simulink library "security_block"  (R2023b)
settings: Solver=VariableStepAuto  StartTime=0.0  StopTime=10.0  RelTol=1e-3
settings Model: Creator=mueller.chris-it22  LastModifiedBy=kilia

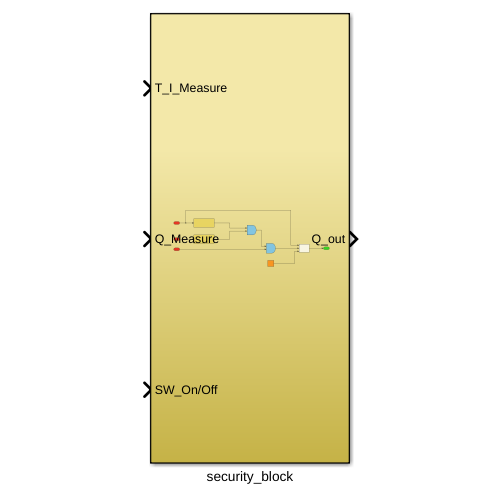
[thumbnail: Simulink's stored preview of the top-level diagram]
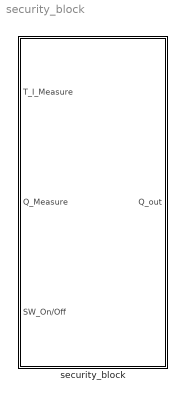
== system security_block ==
  security_block : Subsystem

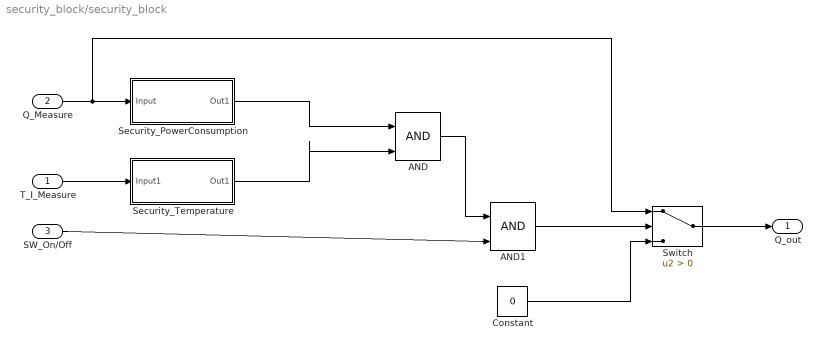
== system security_block/security_block ==
  T_I_Measure : Inport
  Q_Measure : Inport  Port=2
  SW_On/Off : Inport  Port=3
  AND : Logic  IconShape=distinctive  AllPortsSameDT=off  OutDataTypeStr=boolean
  AND1 : Logic  IconShape=distinctive  AllPortsSameDT=off  OutDataTypeStr=boolean
  Constant : Constant  Value=0
  Security_PowerConsumption : Subsystem
  Security_Temperature : Subsystem
  Switch : Switch  Criteria=u2 > Threshold  SaturateOnIntegerOverflow=off  InputSameDT=off
  Q_out : Outport
  wires:
  Q_Measure/1 -> Switch/1, Security_PowerConsumption/1(Input)
  T_I_Measure/1 -> Security_Temperature/1(Input1)
  Security_PowerConsumption/1(Out1) -> AND/1
  Security_Temperature/1(Out1) -> AND/2
  AND1/1 -> Switch/2
  SW_On/Off/1 -> AND1/2
  Switch/1 -> Q_out/1
  Constant/1 -> Switch/3
  AND/1 -> AND1/1

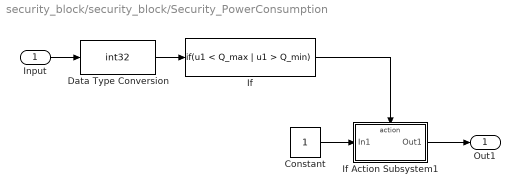
== system security_block/security_block/Security_PowerConsumption ==
  Input : Inport
  Constant : Constant
  Data Type Conversion : DataTypeConversion  OutDataTypeStr=int32  SaturateOnIntegerOverflow=off  RndMeth=Floor
  If : If  IfExpression=u1 < Q_max | u1 > Q_min  ShowElse=off
  If Action Subsystem1 : Subsystem  TreatAsAtomicUnit=on
  Out1 : Outport
  wires:
  Input/1 -> Data Type Conversion/1
  If/1 -> If Action Subsystem1/Action
  If Action Subsystem1/1(Out1) -> Out1/1
  Constant/1 -> If Action Subsystem1/1(In1)
  Data Type Conversion/1 -> If/1

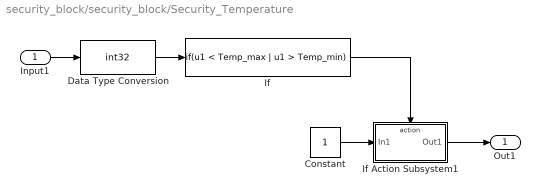
== system security_block/security_block/Security_Temperature ==
  Input1 : Inport
  Constant : Constant
  Data Type Conversion : DataTypeConversion  OutDataTypeStr=int32  SaturateOnIntegerOverflow=off  RndMeth=Floor
  If : If  IfExpression=u1 < Temp_max | u1 > Temp_min  ShowElse=off
  If Action Subsystem1 : Subsystem  TreatAsAtomicUnit=on
  Out1 : Outport
  wires:
  Constant/1 -> If Action Subsystem1/1(In1)
  If Action Subsystem1/1(Out1) -> Out1/1
  If/1 -> If Action Subsystem1/Action
  Data Type Conversion/1 -> If/1
  Input1/1 -> Data Type Conversion/1

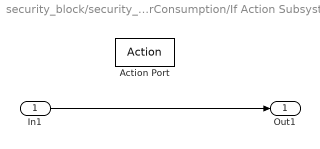
== system security_block/security_block/Security_PowerConsumption/If Action Subsystem1 ==
  In1 : Inport
  Action Port : ActionPort
  Out1 : Outport
  wires:
  In1/1 -> Out1/1

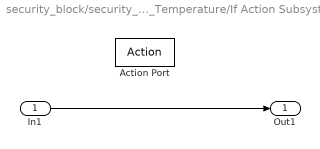
== system security_block/security_block/Security_Temperature/If Action Subsystem1 ==
  In1 : Inport
  Action Port : ActionPort
  Out1 : Outport
  wires:
  In1/1 -> Out1/1
